simulink model "sim_elicottero_filtri"  (R2025b)
settings: Solver=ode4  StartTime=0.0  StopTime=15.0  FixedStep=0.001  RelTol=1e-3
values from neighbouring files (symbols this model uses):
  den_2nd = [1, 2*zeta*omega_n, omega_n^2]    [gen_dataset.m]
  den_pade = [tau_d/2, 1]    [gen_dataset.m]
  dt = log_vars.dt    [ekf_ukf.m]    (also in gen_dataset.m = 0.001)
  log_vars =     [EKF_smoother_data.mat]    (also in dataset_elicottero.mat)
  num_2nd = omega_n^2    (= 900)    [gen_dataset.m]
  num_pade = [-tau_d/2, 1]    [gen_dataset.m]
  p_hat = p    [gen_dataset.m]
  Q = diag([1e-5, 1e-3, 1e-5, 1e-3])    [ekf_ukf.m]    (also in gen_dataset.m = diag([)
  R = diag([0.05, 0.01])    [ekf_ukf.m]    (also in gen_dataset.m = diag([std_v_acc^2, std_v_mag^2, std_v_mag^2]))
  u_0 = [0; 0]    [gen_dataset.m]
  x_0 = [0.1; 0; 0.1; 0]    [gen_dataset.m]
libraries: simulink x4
settings Model: Creator=39345  LastModifiedBy=39345

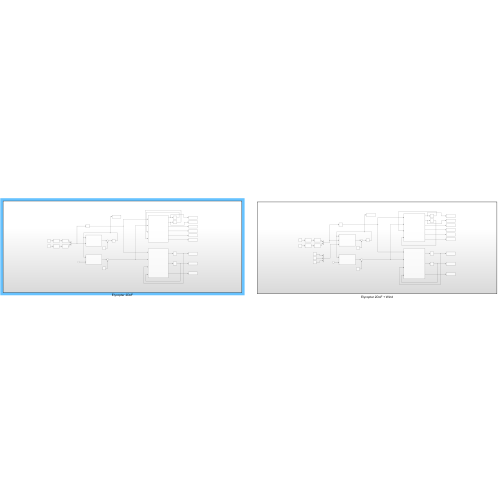
[thumbnail: Simulink's stored preview of the top-level diagram]
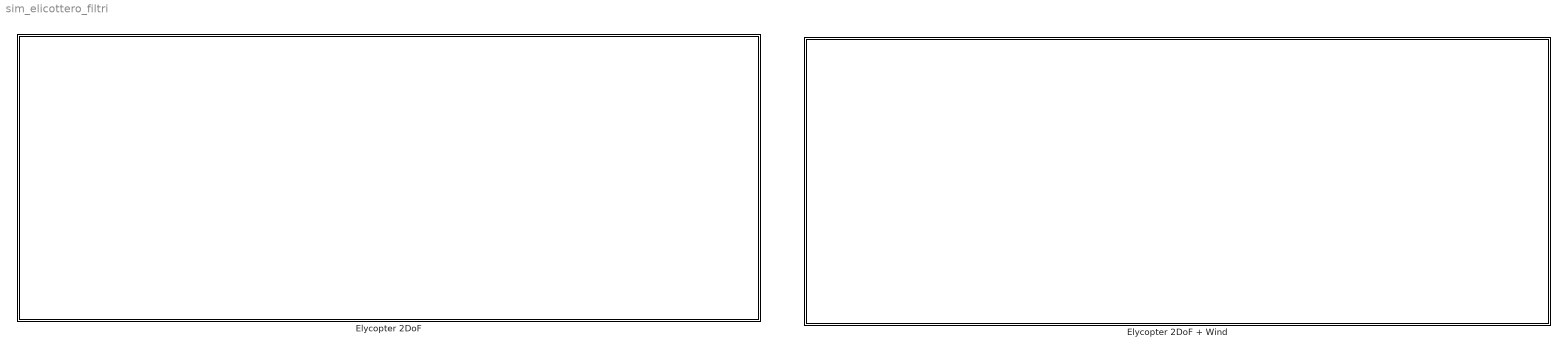
== system sim_elicottero_filtri ==
  Elycopter 2DoF : Subsystem
  Elycopter 2DoF + Wind : Subsystem

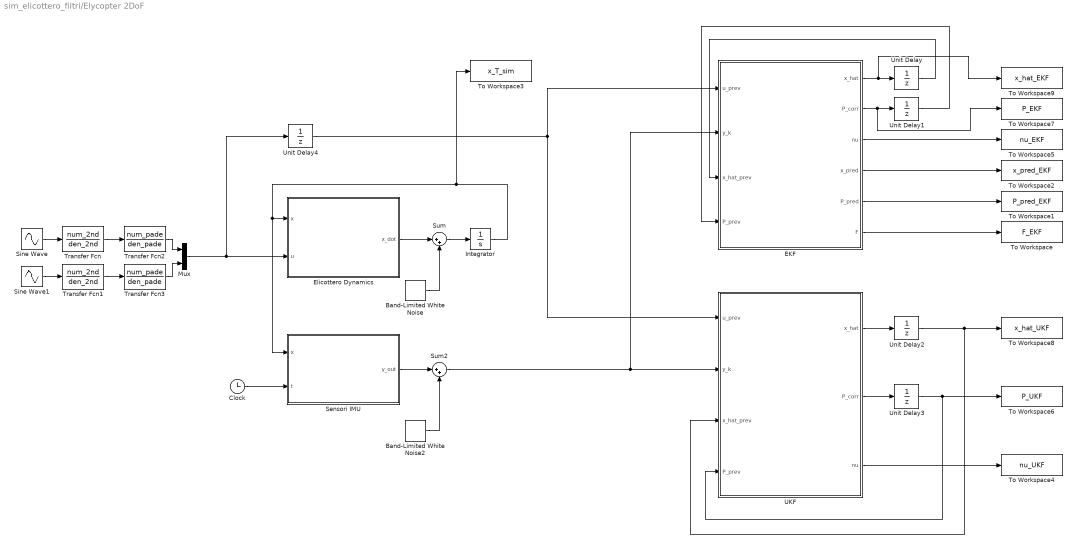
== system sim_elicottero_filtri/Elycopter 2DoF ==
  Band-Limited White Noise : simulink/Sources/Band-Limited White Noise  Cov=[0, 0.0025*dt, 0, 0.0025*dt]  Ts=dt  seed=[23341]
  Band-Limited White Noise2 : simulink/Sources/Band-Limited White Noise  Cov=[(0.2^2)*dt, (0.05^2)*0.01, (0.05^2)*0.01]  Ts=dt  seed=[23341]
  Clock : Clock
  EKF : MATLAB Function  TreatAsAtomicUnit=on
  Elicottero Dynamics : MATLAB Function  TreatAsAtomicUnit=on
  Integrator : Integrator  InitialCondition=x_0
  Mux : Mux  Inputs=2
  Sensori IMU : MATLAB Function  TreatAsAtomicUnit=on
  Sine Wave : Sin  Amplitude=0.5  Frequency=2  SampleTime=0
  Sine Wave1 : Sin  Amplitude=0.3  Frequency=1.5  Phase=pi/2  SampleTime=0
  Sum : Sum  Inputs=|++
  Sum2 : Sum  Inputs=|++
  To Workspace : ToWorkspace  VariableName=F_EKF  SaveFormat=Timeseries  SampleTime=-1
  To Workspace1 : ToWorkspace  VariableName=P_pred_EKF  SaveFormat=Timeseries  SampleTime=-1
  To Workspace2 : ToWorkspace  VariableName=x_pred_EKF  SaveFormat=Timeseries  SampleTime=-1
  To Workspace3 : ToWorkspace  VariableName=x_T_sim  SaveFormat=Timeseries  SampleTime=-1
  To Workspace4 : ToWorkspace  VariableName=nu_UKF  SaveFormat=Timeseries  SampleTime=-1
  To Workspace5 : ToWorkspace  VariableName=nu_EKF  SaveFormat=Timeseries  SampleTime=-1
  To Workspace6 : ToWorkspace  VariableName=P_UKF  SaveFormat=Timeseries  SampleTime=-1
  To Workspace7 : ToWorkspace  VariableName=P_EKF  SaveFormat=Timeseries  SampleTime=-1
  To Workspace8 : ToWorkspace  VariableName=x_hat_UKF  SaveFormat=Timeseries  SampleTime=-1
  To Workspace9 : ToWorkspace  VariableName=x_hat_EKF  SaveFormat=Timeseries  SampleTime=-1
  Transfer Fcn : TransferFcn  Numerator=num_2nd  Denominator=den_2nd
  Transfer Fcn1 : TransferFcn  Numerator=num_2nd  Denominator=den_2nd
  Transfer Fcn2 : TransferFcn  Numerator=num_pade  Denominator=den_pade
  Transfer Fcn3 : TransferFcn  Numerator=num_pade  Denominator=den_pade
  UKF : MATLAB Function  TreatAsAtomicUnit=on
  Unit Delay : UnitDelay  InitialCondition=log_vars.x_hat_0  SampleTime=-1  HasFrameUpgradeWarning=on
  Unit Delay1 : UnitDelay  InitialCondition=log_vars.P_0  SampleTime=dt  HasFrameUpgradeWarning=on
  Unit Delay2 : UnitDelay  InitialCondition=log_vars.x_hat_0  SampleTime=-1  HasFrameUpgradeWarning=on
  Unit Delay3 : UnitDelay  InitialCondition=log_vars.P_0  SampleTime=dt  HasFrameUpgradeWarning=on
  Unit Delay4 : UnitDelay  InitialCondition=u_0  SampleTime=dt  HasFrameUpgradeWarning=on
  wires:
  Sine Wave1/1 -> Transfer Fcn1/1
  UKF/2(P_corr) -> Unit Delay3/1
  EKF/5(P_pred) -> To Workspace1/1
  EKF/4(x_pred) -> To Workspace2/1
  Unit Delay2/1 -> To Workspace8/1, UKF/3(x_hat_prev)
  Transfer Fcn1/1 -> Transfer Fcn3/1
  Integrator/1 -> To Workspace3/1, Sensori IMU/1(x), Elicottero Dynamics/1(x)
  Mux/1 -> Unit Delay4/1, Elicottero Dynamics/2(u)
  Unit Delay3/1 -> To Workspace6/1, UKF/4(P_prev)
  Band-Limited White Noise2/1 -> Sum2/2
  UKF/3(nu) -> To Workspace4/1
  Unit Delay/1 -> EKF/3(x_hat_prev)
  Sum2/1 -> EKF/2(y_k), UKF/2(y_k)
  Sensori IMU/1(y_out) -> Sum2/1
  Unit Delay4/1 -> EKF/1(u_prev), UKF/1(u_prev)
  Transfer Fcn/1 -> Transfer Fcn2/1
  Transfer Fcn3/1 -> Mux/2
  Transfer Fcn2/1 -> Mux/1
  Unit Delay1/1 -> EKF/4(P_prev)
  EKF/6(F) -> To Workspace/1
  Band-Limited White Noise/1 -> Sum/2
  Elicottero Dynamics/1(x_dot) -> Sum/1
  EKF/2(P_corr) -> To Workspace7/1, Unit Delay1/1
  Sine Wave/1 -> Transfer Fcn/1
  EKF/3(nu) -> To Workspace5/1
  EKF/1(x_hat) -> To Workspace9/1, Unit Delay/1
  UKF/1(x_hat) -> Unit Delay2/1
  Sum/1 -> Integrator/1
  Clock/1 -> Sensori IMU/2(t)

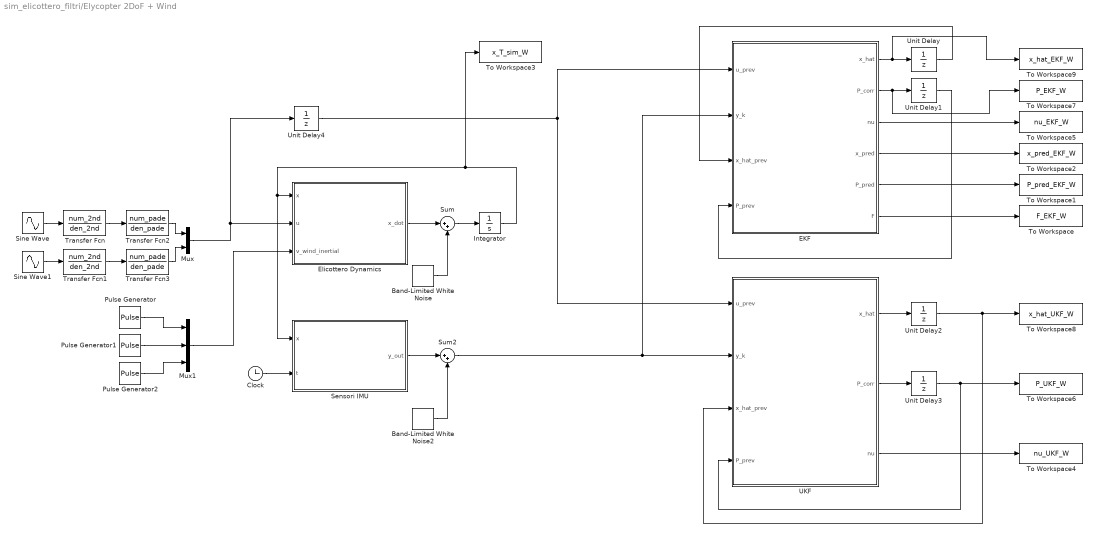
== system sim_elicottero_filtri/Elycopter 2DoF + Wind ==
  Band-Limited White Noise : simulink/Sources/Band-Limited White Noise  Cov=[0, 0.0025*dt, 0, 0.0025*dt]  Ts=dt  seed=[23341]
  Band-Limited White Noise2 : simulink/Sources/Band-Limited White Noise  Cov=[(0.2^2)*dt, (0.05^2)*0.01, (0.05^2)*0.01]  Ts=dt  seed=[23341]
  Clock : Clock
  EKF : MATLAB Function  TreatAsAtomicUnit=on
  Elicottero Dynamics : MATLAB Function  TreatAsAtomicUnit=on
  Integrator : Integrator  InitialCondition=x_0
  Mux : Mux  Inputs=2
  Mux1 : Mux  Inputs=3
  Pulse Generator : DiscretePulseGenerator  Period=10  PulseWidth=5  PhaseDelay=5
  Pulse Generator1 : DiscretePulseGenerator  Period=10  PulseWidth=5  PhaseDelay=5
  Pulse Generator2 : DiscretePulseGenerator  Period=10  PulseWidth=5  PhaseDelay=5
  Sensori IMU : MATLAB Function  TreatAsAtomicUnit=on
  Sine Wave : Sin  Amplitude=0.5  Frequency=2  SampleTime=0
  Sine Wave1 : Sin  Amplitude=0.3  Frequency=1.5  Phase=pi/2  SampleTime=0
  Sum : Sum  Inputs=|++
  Sum2 : Sum  Inputs=|++
  To Workspace : ToWorkspace  VariableName=F_EKF_W  SaveFormat=Timeseries  SampleTime=-1
  To Workspace1 : ToWorkspace  VariableName=P_pred_EKF_W  SaveFormat=Timeseries  SampleTime=-1
  To Workspace2 : ToWorkspace  VariableName=x_pred_EKF_W  SaveFormat=Timeseries  SampleTime=-1
  To Workspace3 : ToWorkspace  VariableName=x_T_sim_W  SaveFormat=Timeseries  SampleTime=-1
  To Workspace4 : ToWorkspace  VariableName=nu_UKF_W  SaveFormat=Timeseries  SampleTime=-1
  To Workspace5 : ToWorkspace  VariableName=nu_EKF_W  SaveFormat=Timeseries  SampleTime=-1
  To Workspace6 : ToWorkspace  VariableName=P_UKF_W  SaveFormat=Timeseries  SampleTime=-1
  To Workspace7 : ToWorkspace  VariableName=P_EKF_W  SaveFormat=Timeseries  SampleTime=-1
  To Workspace8 : ToWorkspace  VariableName=x_hat_UKF_W  SaveFormat=Timeseries  SampleTime=-1
  To Workspace9 : ToWorkspace  VariableName=x_hat_EKF_W  SaveFormat=Timeseries  SampleTime=-1
  Transfer Fcn : TransferFcn  Numerator=num_2nd  Denominator=den_2nd
  Transfer Fcn1 : TransferFcn  Numerator=num_2nd  Denominator=den_2nd
  Transfer Fcn2 : TransferFcn  Numerator=num_pade  Denominator=den_pade
  Transfer Fcn3 : TransferFcn  Numerator=num_pade  Denominator=den_pade
  UKF : MATLAB Function  TreatAsAtomicUnit=on
  Unit Delay : UnitDelay  InitialCondition=log_vars.x_hat_0  SampleTime=-1  HasFrameUpgradeWarning=on
  Unit Delay1 : UnitDelay  InitialCondition=log_vars.P_0  SampleTime=dt  HasFrameUpgradeWarning=on
  Unit Delay2 : UnitDelay  InitialCondition=log_vars.x_hat_0  SampleTime=-1  HasFrameUpgradeWarning=on
  Unit Delay3 : UnitDelay  InitialCondition=log_vars.P_0  SampleTime=dt  HasFrameUpgradeWarning=on
  Unit Delay4 : UnitDelay  InitialCondition=u_0  SampleTime=dt  HasFrameUpgradeWarning=on
  wires:
  Sine Wave1/1 -> Transfer Fcn1/1
  UKF/2(P_corr) -> Unit Delay3/1
  EKF/5(P_pred) -> To Workspace1/1
  EKF/4(x_pred) -> To Workspace2/1
  Unit Delay2/1 -> To Workspace8/1, UKF/3(x_hat_prev)
  Transfer Fcn1/1 -> Transfer Fcn3/1
  Integrator/1 -> To Workspace3/1, Sensori IMU/1(x), Elicottero Dynamics/1(x)
  Mux/1 -> Unit Delay4/1, Elicottero Dynamics/2(u)
  Unit Delay3/1 -> To Workspace6/1, UKF/4(P_prev)
  Band-Limited White Noise2/1 -> Sum2/2
  UKF/3(nu) -> To Workspace4/1
  Unit Delay/1 -> EKF/3(x_hat_prev)
  Sum2/1 -> EKF/2(y_k), UKF/2(y_k)
  Sensori IMU/1(y_out) -> Sum2/1
  Unit Delay4/1 -> EKF/1(u_prev), UKF/1(u_prev)
  Transfer Fcn/1 -> Transfer Fcn2/1
  Transfer Fcn3/1 -> Mux/2
  Transfer Fcn2/1 -> Mux/1
  Unit Delay1/1 -> EKF/4(P_prev)
  EKF/6(F) -> To Workspace/1
  Band-Limited White Noise/1 -> Sum/2
  Elicottero Dynamics/1(x_dot) -> Sum/1
  EKF/2(P_corr) -> To Workspace7/1, Unit Delay1/1
  Sine Wave/1 -> Transfer Fcn/1
  EKF/3(nu) -> To Workspace5/1
  EKF/1(x_hat) -> To Workspace9/1, Unit Delay/1
  UKF/1(x_hat) -> Unit Delay2/1
  Sum/1 -> Integrator/1
  Mux1/1 -> Elicottero Dynamics/3(v_wind_inertial)
  Pulse Generator/1 -> Mux1/1
  Pulse Generator1/1 -> Mux1/2
  Pulse Generator2/1 -> Mux1/3
  Clock/1 -> Sensori IMU/2(t)

== matlab function sim_elicottero_filtri/Elycopter 2DoF + Wind/Sensori IMU ==
  data: x input; y_out output; p parameter; t input
function y_out = sensori_imu(x, p, t)
    % ESTRAZIONE STATI RILEVANTI
    alpha = x(1);
    beta = x(3);
    
    % EQUAZIONI DEI SENSORI (Misure ideali)
    % 1. Accelerometro asse X (misura per alpha)
    y_acc = -p.g * sin(alpha);
    
    % 2. Magnetometro asse X e Y (misura per beta)
    mx = cos(alpha)*cos(beta);
    my = -sin(beta);

    y_out = [y_acc;
            mx;
            my];
    
    % ========================================================
    % LOGICA MULTI-RATE (Mascheramento dati mancanti)
    % ========================================================
    % Supponiamo che l'accelerometro (y_acc) lavori ad alta frequenza 
    % e sia sempre disponibile (quindi non lo tocchiamo).
    % Supponiamo che il magnetometro (y_mag) lavori a 10 Hz (un dato ogni 0.1 s).
    
    Tc_mag = 0.01; % Tempo di campionamento del sensore lento [secondi]
    tol = 1e-4;   % Tolleranza per gli arrotondamenti numerici di Simulink
    
    % Calcolo il resto della divisione tra il tempo attuale e il Tc del sensore
    resto = mod(t, Tc_mag);
    
    % Se il tempo attuale NON è un multiplo esatto di 0.1 secondi
    if resto > tol && (Tc_mag - resto) > tol
        % Il magnetometro non ha ancora prodotto un nuovo dato.
        % Sostituisco la seconda misura con Not a Number (NaN).
        y_out(2) = NaN; 
        y_out(3) = NaN;
    end
end

== matlab function sim_elicottero_filtri/Elycopter 2DoF + Wind/UKF ==
  data: u_prev input; x_hat output; y_k input; x_hat_prev input; P_prev input; P_corr output; nu output; Q parameter; R parameter; dt parameter; p_hat parameter
function [x_hat, P_corr, nu] = UKF_Filter(u_prev, y_k, x_hat_prev, P_prev, Q, R, dt, p_hat)
    
    % 1. Predizione UKF
    [x_pred, P_pred] = UnscentedTransform_F(x_hat_prev, P_prev, Q, dt, u_prev, p_hat);
    
    % 2. Correzione UKF
    [hat_y, S, Pxy] = UnscentedTransform_H(x_pred, P_pred, R, p_hat);
    
    % Logica Multi-rate
    idx_validi = ~isnan(y_k); 
    
    % Inizializzo default (come nell'EKF)
    x_hat = x_pred;
    P_corr = P_pred;
    nu = [0; 0; 0];
    
    if any(idx_validi)
        % Ritaglio solo i dati dei sensori attivi
        y_k_valid   = y_k(idx_validi);
        hat_y_valid = hat_y(idx_validi);
        
        S_valid   = S(idx_validi, idx_validi);
        Pxy_valid = Pxy(:, idx_validi); % Mantengo tutte le righe degli stati, ritaglio le colonne
        
        
        nu_valid = y_k_valid - hat_y_valid;
        
        % Salvo l'innovazione per i log
        nu(idx_validi) = nu_valid;

        % 3. DISTANZA DI MAHALANOBIS (Gating)
        D2 = nu_valid' * (S_valid \ nu_valid); 
        
        % Imposto la soglia Chi-Quadro al 95% in base a quanti sensori stanno parlando
        gradi_liberta = sum(idx_validi);
        if gradi_liberta == 1
            soglia = 3.84;
        else
            soglia = 7.81;
        end
        
        % 4. Aggiornamento dello Stato (solo se la misura è plausibile)
        if D2 < soglia
            L = Pxy_valid / S_valid;
            x_hat = x_pred + L * nu_valid;
            P_corr = P_pred - L * S_valid * L';            
        else
            % Outlier rilevato dal Mahalanobis! Ignoro la misura e tengo la predizione
            % (x_hat e P_corr restano x_pred e P_pred come inizializzato sopra)
        end
    end
end

% --- Funzioni Locali ---
function [mean_f, cov_f] = UnscentedTransform_F(x, P, Q, dt, u, p_hat)
    n = length(x);
    alpha = 1e-2; kappa = 0; beta = 2;
    lambda = alpha^2 * (n + kappa) - n;
    w_m = [lambda/(n+lambda), repmat(1/(2*(n+lambda)), 1, 2*n)];
    w_c = w_m; w_c(1) = w_c(1) + (1 - alpha^2 + beta);
    
    [U, S_mat, ~] = svd(P);
    GAMMA = U * sqrt(S_mat);
    
    sigmas = zeros(n, 2*n+1);
    sigmas(:,1) = x;
    for i = 1:n
        sigmas(:, i+1)   = x + sqrt(n+lambda)*GAMMA(:,i);
        sigmas(:, i+1+n) = x - sqrt(n+lambda)*GAMMA(:,i);
    end
    
    sigmas_f = zeros(n, 2*n+1);
    for i = 1:size(sigmas, 2)
        al = sigmas(1,i); al_d = sigmas(2,i); be = sigmas(3,i); be_d = sigmas(4,i);
        J_b = p_hat.J_y * sin(al)^2 + (p_hat.J_z + p_hat.m*p_hat.l^2)*cos(al)^2 + p_hat.I_b;

        % 1. Velocità angolare in Body
        omega_body = [-be_d * sin(al); al_d; be_d * cos(al)];
        % 2. Velocità lineare del corpo (v = omega x r)
        v_body = cross(omega_body, [p_hat.l; 0; 0]);
        % 3. Velocità relativa (il filtro assume vento esterno nullo)
        v_rel_body = -v_body;
        v_rel_norm = norm(v_rel_body);
        
        % 4. Forza aerodinamica (segno positivo corretto)
        F_drag_body = 0.5 * p_hat.rho * p_hat.Cd_A .* v_rel_body * v_rel_norm;
        
        % 5. Coppie di drag (segni corretti da prodotto vettoriale)
        tau_drag_alpha = -p_hat.l * F_drag_body(3);
        tau_drag_beta  =  p_hat.l * F_drag_body(2);

        al_dd = (-p_hat.c_alpha*al_d - p_hat.m*p_hat.g*p_hat.l*sin(al) + p_hat.l*u(1)*cos(be) + p_hat.eps_p*p_hat.l*u(2)*sin(be) + tau_drag_alpha) / p_hat.J_alpha;
        be_dd = (-p_hat.c_beta*be_d + p_hat.l*u(2)*cos(al) + p_hat.eps_y*p_hat.l*u(1)*sin(al) + tau_drag_beta) / J_b;
        sigmas_f(:,i) = [al + dt*al_d; al_d + dt*al_dd; be + dt*be_d; be_d + dt*be_dd];
    end
    
    mean_f = sigmas_f * w_m';
    tilde_f = sigmas_f - mean_f;
    cov_f = (tilde_f .* w_c) * tilde_f' + Q;
end

function [mean_h, cov_h, cross_cov] = UnscentedTransform_H(x, P, R, p_hat)
    n = length(x);
    alpha = 5e-2; kappa = 0; beta = 2;
    lambda = alpha^2 * (n + kappa) - n;
    
    w_m = [lambda/(n+lambda), repmat(1/(2*(n+lambda)), 1, 2*n)];
    w_c = w_m; w_c(1) = w_c(1) + (1 - alpha^2 + beta);
    
    [U, S_mat, ~] = svd(P);
    GAMMA = U * sqrt(S_mat);
    
    sigmas = zeros(n, 2*n+1);
    sigmas(:,1) = x;
    for i = 1:n
        sigmas(:, i+1)   = x + sqrt(n+lambda)*GAMMA(:,i);
        sigmas(:, i+1+n) = x - sqrt(n+lambda)*GAMMA(:,i);
    end
    
    sigmas_h = zeros(3, 2*n+1);
    for i = 1:size(sigmas, 2)
        sigmas_h(1,i) = -p_hat.g * sin(sigmas(1,i));
        sigmas_h(2,i) = cos(sigmas(1,i)) * cos(sigmas(3,i));
        sigmas_h(3,i) = -sin(sigmas(3,i));
    end
    
    mean_h = sigmas_h * w_m';
    tilde_h = sigmas_h - mean_h;
    cov_h = (tilde_h .* w_c) * tilde_h' + R;
    
    tilde_x = sigmas - x;
    cross_cov = (tilde_x .* w_c) * tilde_h';
end

== matlab function sim_elicottero_filtri/Elycopter 2DoF/Sensori IMU ==
  settings: sampleTime=dt
  data: x input; y_out output; p parameter; t input
function y_out = sensori_imu(x, p, t)
    % ESTRAZIONE STATI RILEVANTI
    alpha = x(1);
    beta = x(3);
    
    % EQUAZIONI DEI SENSORI (Misure ideali)
    % 1. Accelerometro asse X (misura per alpha)
    y_acc = -p.g * sin(alpha);
    
    % 2. Magnetometro asse X e Y (misura per beta)
    mx = cos(alpha)*cos(beta);
    my = -sin(beta);

    y_out = [y_acc;
            mx;
            my];
    
    % ========================================================
    % LOGICA MULTI-RATE (Mascheramento dati mancanti)
    % ========================================================
    % Supponiamo che l'accelerometro (y_acc) lavori ad alta frequenza 
    % e sia sempre disponibile (quindi non lo tocchiamo).
    % Supponiamo che il magnetometro (y_mag) lavori a 10 Hz (un dato ogni 0.1 s).
    
    Tc_mag = 0.01; % Tempo di campionamento del sensore lento [secondi]
    tol = 1e-4;   % Tolleranza per gli arrotondamenti numerici di Simulink
    
    % Calcolo il resto della divisione tra il tempo attuale e il Tc del sensore
    resto = mod(t, Tc_mag);
    
    % Se il tempo attuale NON è un multiplo esatto di 0.1 secondi
    if resto > tol && (Tc_mag - resto) > tol
        % Il magnetometro non ha ancora prodotto un nuovo dato.
        % Sostituisco la seconda misura con Not a Number (NaN).
        y_out(2) = NaN; 
        y_out(3) = NaN;
    end
end

== matlab function sim_elicottero_filtri/Elycopter 2DoF/Elicottero Dynamics ==
  data: x input; u input; x_dot output; p parameter
function x_dot = elicottero_dynamics(x, u, p)
    % ESTRAZIONE STATI
    alpha = x(1);
    alpha_dot = x(2);
    beta = x(3);
    beta_dot = x(4);
    
    % ESTRAZIONE INGRESSI
    F1 = u(1);
    F2 = u(2);
                 
    % 1. Vettore velocità angolare nel sistema Body (omega_B)
    % Il Pitch (alpha_dot) ruota attorno all'asse Y_body.
    % Lo Yaw (beta_dot) ruota attorno all'asse Z_inerziale, che proiettato in Body diventa [-sin(alpha); 0; cos(alpha)]
    omega_body = [-beta_dot * sin(alpha); 
                   alpha_dot; 
                   beta_dot * cos(alpha)];
                   
    % 2. Vettore posizione del centro aerodinamico (i rotori a distanza l sull'asse X_body)
    r_cp = [p.l; 0; 0];
    
    % 3. Velocità lineare del corpo dovuta alla rotazione (v = omega x r)
    v_corpo_body = cross(omega_body, r_cp); 
    % (Il risultato analitico sarà: [0; p.l * beta_dot * cos(alpha); -p.l * alpha_dot])
    
    
    % 5. VELOCITÀ RELATIVA VERA (Vento esterno - Velocità del corpo)
    v_rel_body  = - v_corpo_body; 
    v_rel_norm  = norm(v_rel_body);
    
    % Calcolo Forze Aerodinamiche
    % NOTA: Per pulizia del codice, in futuro potresti spostare rho e Cd_A 
    % all'interno della struct dei parametri 'p'
    rho = 1.225; % Densità dell'aria [kg/m^3]
    Cd_A = [0.1
            0.1
            0.2]; % Prodotto Cd * Area per gli assi [X; Y; Z]
    % Bracci da $0.25$ e $0.30$ m: Sono lunghezze tipiche dei bracci di un 
    % elicottero didattico da laboratorio a 2 gradi di libertà, come i 
    % classici modelli Quanser Aero o i TRMS (Twin Rotor MIMO System)
    
    F_drag_body = 0.5 * rho * Cd_A .* v_rel_body * v_rel_norm;
    
    % Calcolo Coppie di Disturbo
    % Assumiamo che la forza aerodinamica agisca con braccio pari a p.l
    tau_wind_alpha = -F_drag_body(3) * p.l; % Forza verticale genera coppia di pitch
    tau_wind_beta  = F_drag_body(2) * p.l; % Forza laterale genera coppia di yaw
    
    % DINAMICA: Inerzia variabile di yaw
    J_beta = p.J_y * sin(alpha)^2 + (p.J_z + p.m*p.l^2)*cos(alpha)^2 + p.I_b;
    
    % EQUAZIONI DEL MOTO (Accelerazioni)
    % I momenti del vento sono sommati ai momenti generati dai motori
    alpha_ddot = (-p.c_alpha*alpha_dot - p.m*p.g*p.l*sin(alpha) + p.l*F1*cos(beta) + p.eps_p*p.l*F2*sin(beta) + tau_wind_alpha) / p.J_alpha;
    beta_ddot  = (-p.c_beta*beta_dot + p.l*F2*cos(alpha) + p.eps_y*p.l*F1*sin(alpha) + tau_wind_beta) / J_beta;
    
    
    % USCITA: Vettore colonna delle derivate dello stato
    x_dot = [alpha_dot; alpha_ddot; beta_dot; beta_ddot];
end

== matlab function sim_elicottero_filtri/Elycopter 2DoF/EKF ==
  data: u_prev input; x_hat output; y_k input; x_hat_prev input; P_prev input; P_corr output; nu output; Q parameter; R parameter; dt parameter; p_hat parameter; x_pred output; P_pred output; F output
function [x_hat, P_corr, nu, x_pred, P_pred, F] = EKF_Filter(u_prev, y_k, x_hat_prev, P_prev, Q, R, dt, p_hat)
    % ========================================================
    % 1. FASE DI PREDIZIONE
    % ========================================================
    alpha = x_hat_prev(1); alpha_dot = x_hat_prev(2); 
    beta = x_hat_prev(3);  beta_dot = x_hat_prev(4);
    F1 = u_prev(1); F2 = u_prev(2);

    rho = 1.225; % Densità dell'aria [kg/m^3]
    Cd_A = [0.5; 0.6; 1.2]; % Prodotto Cd * Area per gli assi [X; Y; Z]
    
    J_beta = p_hat.J_y * sin(alpha)^2 + (p_hat.J_z + p_hat.m*p_hat.l^2)*cos(alpha)^2 + p_hat.I_b;

    omega_body = [-beta_dot * sin(alpha); alpha_dot; beta_dot * cos(alpha)];
    v_corpo_body = cross(omega_body, [p_hat.l; 0; 0]);
    v_rel_body = -v_corpo_body; % Il filtro assume vento esterno nullo
    v_rel_norm = norm(v_rel_body);
    
    F_drag_body = 0.5 * rho * Cd_A .* v_rel_body * v_rel_norm;
    tau_drag_alpha = -F_drag_body(3) * p_hat.l;
    tau_drag_beta  = F_drag_body(2) * p_hat.l;

    alpha_ddot = (-p_hat.c_alpha*alpha_dot - p_hat.m*p_hat.g*p_hat.l*sin(alpha) + p_hat.l*F1*cos(beta) + p_hat.eps_p*p_hat.l*F2*sin(beta) + tau_drag_alpha) / p_hat.J_alpha;
    beta_ddot  = (-p_hat.c_beta*beta_dot + p_hat.l*F2*cos(alpha) + p_hat.eps_y*p_hat.l*F1*sin(alpha) + tau_drag_beta) / J_beta;
    
    x_pred = [alpha + dt * alpha_dot;
              alpha_dot + dt * alpha_ddot;
              beta + dt * beta_dot;
              beta_dot + dt * beta_ddot];

    % Jacobiano numerico F
    [F, ~] = jacobiani_analitici(x_hat_prev(1), x_hat_prev(2), x_hat_prev(3), x_hat_prev(4), ...
                           u_prev(1), u_prev(2), dt, rho, ...
                           p_hat.m, p_hat.l, p_hat.g, p_hat.J_y, p_hat.J_z, p_hat.I_b, p_hat.J_alpha, ...
                           p_hat.c_alpha, p_hat.c_beta, p_hat.eps_p, p_hat.eps_y, ...
                           Cd_A(1), Cd_A(2), Cd_A(3));

    P_pred = F * P_prev * F' + Q;

% ========================================================
    % 2. FASE DI CORREZIONE
    % ========================================================
    % Calcolo la misura attesa completa
    hat_y = [-p_hat.g * sin(x_pred(1));
             cos(x_pred(1)) * cos(x_pred(3));
             -sin(x_pred(3))];
    
    % Calcolo il Jacobiano H completo
    [~, H] = jacobiani_analitici(x_pred(1), x_pred(2), x_pred(3), x_pred(4), ...
                           u_prev(1), u_prev(2), dt, rho, ...
                           p_hat.m, p_hat.l, p_hat.g, p_hat.J_y, p_hat.J_z, p_hat.I_b, p_hat.J_alpha, ...
                           p_hat.c_alpha, p_hat.c_beta, p_hat.eps_p, p_hat.eps_y, ...
                           Cd_A(1), Cd_A(2), Cd_A(3));
     
    % Trovo quali sensori hanno inviato un dato valido in questo istante
    % (idx_validi sarà un vettore logico, es: [1; 0] se è arrivato solo il sensore 1)
    idx_validi = ~isnan(y_k); 
    
    % Inizializzo le uscite di default (se nessun sensore parla, tengo la predizione)
    x_hat = x_pred;
    P_corr = P_pred;
    nu = [0; 0; 0]; % Innovazione nulla di default
    
    if any(idx_validi) % Se almeno un sensore ha un dato nuovo
        
        % 1. "RitAGLIO" i vettori e le matrici tenendo solo le righe dei sensori attivi
        y_k_valid   = y_k(idx_validi);
        hat_y_valid = hat_y(idx_validi);
        H_valid     = H(idx_validi, :);
        
        % Ritaglio anche la matrice R (rumore di misura) per togliere il sensore inattivo
        R_valid     = R(idx_validi, idx_validi);
        
        % 2. Calcolo Innovazione e Covarianza dell'Innovazione ridimensionate
        nu_valid = y_k_valid - hat_y_valid;
        S = H_valid * P_pred * H_valid' + R_valid;
        
        % 3. DISTANZA DI MAHALANOBIS (Gating)
        D2 = nu_valid' * (S \ nu_valid); 
        
        % Imposto la soglia Chi-Quadro al 95% in base a quanti sensori stanno parlando
        gradi_liberta = sum(idx_validi);
        if gradi_liberta == 1
            soglia = 3.84;
        else
            soglia = 5.99;
        end
        
        % 4. Aggiornamento dello Stato (solo se la misura è plausibile)
        if D2 < soglia
            L = P_pred * H_valid' / S;
            x_hat = x_pred + L * nu_valid;
            P_corr = (eye(4) - L * H_valid) * P_pred;
            
            % Salvo l'innovazione calcolata per i log (lasciando 0 dove mancava il dato)
            nu(idx_validi) = nu_valid; 
        else
            % Outlier rilevato dal Mahalanobis! Ignoro la misura e tengo la predizione
            % (x_hat e P_corr restano x_pred e P_pred come inizializzato sopra)
        end
        
    end
end

== matlab function sim_elicottero_filtri/Elycopter 2DoF/UKF ==
  data: u_prev input; x_hat output; y_k input; x_hat_prev input; P_prev input; P_corr output; nu output; Q parameter; R parameter; dt parameter; p_hat parameter
function [x_hat, P_corr, nu] = UKF_Filter(u_prev, y_k, x_hat_prev, P_prev, Q, R, dt, p_hat)
    
    % 1. Predizione UKF
    [x_pred, P_pred] = UnscentedTransform_F(x_hat_prev, P_prev, Q, dt, u_prev, p_hat);
    
    % 2. Correzione UKF
    [hat_y, S, Pxy] = UnscentedTransform_H(x_pred, P_pred, R, p_hat);
    
    % Logica Multi-rate
    idx_validi = ~isnan(y_k); 
    
    % Inizializzo default (come nell'EKF)
    x_hat = x_pred;
    P_corr = P_pred;
    nu = [0; 0; 0];
    
    if any(idx_validi)
        % Ritaglio solo i dati dei sensori attivi
        y_k_valid   = y_k(idx_validi);
        hat_y_valid = hat_y(idx_validi);
        
        S_valid   = S(idx_validi, idx_validi);
        Pxy_valid = Pxy(:, idx_validi); % Mantengo tutte le righe degli stati, ritaglio le colonne
        
        
        nu_valid = y_k_valid - hat_y_valid;
        
        % Salvo l'innovazione per i log
        nu(idx_validi) = nu_valid;

        % 3. DISTANZA DI MAHALANOBIS (Gating)
        D2 = nu_valid' * (S_valid \ nu_valid); 
        
        % Imposto la soglia Chi-Quadro al 95% in base a quanti sensori stanno parlando
        gradi_liberta = sum(idx_validi);
        if gradi_liberta == 1
            soglia = 3.84;
        else
            soglia = 7.81;
        end
        
        % 4. Aggiornamento dello Stato (solo se la misura è plausibile)
        if D2 < soglia
            L = Pxy_valid / S_valid;
            x_hat = x_pred + L * nu_valid;
            P_corr = P_pred - L * S_valid * L';            
        else
            % Outlier rilevato dal Mahalanobis! Ignoro la misura e tengo la predizione
            % (x_hat e P_corr restano x_pred e P_pred come inizializzato sopra)
        end
    end
end

% --- Funzioni Locali ---
function [mean_f, cov_f] = UnscentedTransform_F(x, P, Q, dt, u, p_hat)
    n = length(x);
    alpha = 1e-2; kappa = 0; beta = 2;
    lambda = alpha^2 * (n + kappa) - n;
    w = [0 0 0];
    w_m = [lambda/(n+lambda), repmat(1/(2*(n+lambda)), 1, 2*n)];
    w_c = w_m; w_c(1) = w_c(1) + (1 - alpha^2 + beta);
    
    [U, S_mat, ~] = svd(P);
    GAMMA = U * sqrt(S_mat);
    
    sigmas = zeros(n, 2*n+1);
    sigmas(:,1) = x;
    for i = 1:n
        sigmas(:, i+1)   = x + sqrt(n+lambda)*GAMMA(:,i);
        sigmas(:, i+1+n) = x - sqrt(n+lambda)*GAMMA(:,i);
    end
    
    sigmas_f = zeros(n, 2*n+1);
    for i = 1:size(sigmas, 2)
        al = sigmas(1,i); al_d = sigmas(2,i); be = sigmas(3,i); be_d = sigmas(4,i);
        J_b = p_hat.J_y * sin(al)^2 + (p_hat.J_z + p_hat.m*p_hat.l^2)*cos(al)^2 + p_hat.I_b;

        % 1. Velocità angolare in Body
        omega_body = [-be_d * sin(al); al_d; be_d * cos(al)];
        % 2. Velocità lineare del corpo (v = omega x r)
        v_body = cross(omega_body, [p_hat.l; 0; 0]);
        % 3. Velocità relativa (il filtro assume vento esterno nullo)
        v_rel_body = -v_body + w;
        v_rel_norm = norm(v_rel_body);
        
        % 4. Forza aerodinamica (segno positivo corretto)
        F_drag_body = 0.5 * p_hat.rho * p_hat.Cd_A .* v_rel_body * v_rel_norm;
        
        % 5. Coppie di drag (segni corretti da prodotto vettoriale)
        tau_drag_alpha = -p_hat.l * F_drag_body(3);
        tau_drag_beta  =  p_hat.l * F_drag_body(2);

        al_dd = (-p_hat.c_alpha*al_d - p_hat.m*p_hat.g*p_hat.l*sin(al) + p_hat.l*u(1)*cos(be) + p_hat.eps_p*p_hat.l*u(2)*sin(be) + tau_drag_alpha) / p_hat.J_alpha;
        be_dd = (-p_hat.c_beta*be_d + p_hat.l*u(2)*cos(al) + p_hat.eps_y*p_hat.l*u(1)*sin(al) + tau_drag_beta) / J_b;
        sigmas_f(:,i) = [al + dt*al_d; al_d + dt*al_dd; be + dt*be_d; be_d + dt*be_dd];
    end
    
    mean_f = sigmas_f * w_m';
    tilde_f = sigmas_f - mean_f;
    cov_f = (tilde_f .* w_c) * tilde_f' + Q;
end

function [mean_h, cov_h, cross_cov] = UnscentedTransform_H(x, P, R, p_hat)
    n = length(x);
    alpha = 5e-2; kappa = 0; beta = 2;
    lambda = alpha^2 * (n + kappa) - n;
    
    w_m = [lambda/(n+lambda), repmat(1/(2*(n+lambda)), 1, 2*n)];
    w_c = w_m; w_c(1) = w_c(1) + (1 - alpha^2 + beta);
    
    [U, S_mat, ~] = svd(P);
    GAMMA = U * sqrt(S_mat);
    
    sigmas = zeros(n, 2*n+1);
    sigmas(:,1) = x;
    for i = 1:n
        sigmas(:, i+1)   = x + sqrt(n+lambda)*GAMMA(:,i);
        sigmas(:, i+1+n) = x - sqrt(n+lambda)*GAMMA(:,i);
    end
    
    sigmas_h = zeros(3, 2*n+1);
    for i = 1:size(sigmas, 2)
        sigmas_h(1,i) = -p_hat.g * sin(sigmas(1,i));
        sigmas_h(2,i) = cos(sigmas(1,i)) * cos(sigmas(3,i));
        sigmas_h(3,i) = -sin(sigmas(3,i));
    end
    
    mean_h = sigmas_h * w_m';
    tilde_h = sigmas_h - mean_h;
    cov_h = (tilde_h .* w_c) * tilde_h' + R;
    
    tilde_x = sigmas - x;
    cross_cov = (tilde_x .* w_c) * tilde_h';
end

== matlab function sim_elicottero_filtri/Elycopter 2DoF + Wind/EKF ==
  data: u_prev input; x_hat output; y_k input; x_hat_prev input; P_prev input; P_corr output; nu output; Q parameter; R parameter; dt parameter; p_hat parameter; x_pred output; P_pred output; F output
function [x_hat, P_corr, nu, x_pred, P_pred, F] = EKF_Filter(u_prev, y_k, x_hat_prev, P_prev, Q, R, dt, p_hat)
    % ========================================================
    % 1. FASE DI PREDIZIONE (predict_EKF)
    % ========================================================
    alpha = x_hat_prev(1); alpha_dot = x_hat_prev(2); 
    beta = x_hat_prev(3);  beta_dot = x_hat_prev(4);
    F1 = u_prev(1); F2 = u_prev(2);

    rho = 1.225; % Densità dell'aria [kg/m^3]
    Cd_A = [0.5; 0.6; 1.2]; % Prodotto Cd * Area per gli assi [X; Y; Z]
    J_beta = p_hat.J_y * sin(alpha)^2 + (p_hat.J_z + p_hat.m*p_hat.l^2)*cos(alpha)^2 + p_hat.I_b;

    omega_body = [-beta_dot * sin(alpha); alpha_dot; beta_dot * cos(alpha)];
    v_body = cross(omega_body, [p_hat.l; 0; 0]);
    v_rel_body = -v_body; % Il filtro assume vento esterno nullo
    v_rel_norm = norm(v_rel_body);
    
    F_drag_body = 0.5 * rho * Cd_A .* v_rel_body * v_rel_norm;
    tau_drag_alpha = -F_drag_body(3) * p_hat.l;
    tau_drag_beta  = F_drag_body(2) * p_hat.l;

    alpha_ddot = (-p_hat.c_alpha*alpha_dot - p_hat.m*p_hat.g*p_hat.l*sin(alpha) + p_hat.l*F1*cos(beta) + p_hat.eps_p*p_hat.l*F2*sin(beta) + tau_drag_alpha) / p_hat.J_alpha;
    beta_ddot  = (-p_hat.c_beta*beta_dot + p_hat.l*F2*cos(alpha) + p_hat.eps_y*p_hat.l*F1*sin(alpha) + tau_drag_beta) / J_beta;
    
    x_pred = [alpha + dt * alpha_dot;
              alpha_dot + dt * alpha_ddot;
              beta + dt * beta_dot;
              beta_dot + dt * beta_ddot];

    % Jacobiano numerico F
    [F, ~] = jacobiani_analitici(x_hat_prev(1), x_hat_prev(2), x_hat_prev(3), x_hat_prev(4), ...
                           u_prev(1), u_prev(2), dt, rho, ...
                           p_hat.m, p_hat.l, p_hat.g, p_hat.J_y, p_hat.J_z, p_hat.I_b, p_hat.J_alpha, ...
                           p_hat.c_alpha, p_hat.c_beta, p_hat.eps_p, p_hat.eps_y, ...
                           Cd_A(1), Cd_A(2), Cd_A(3));

    P_pred = F * P_prev * F' + Q;

    % ========================================================
    % 2. FASE DI CORREZIONE (correct_EKF) - MULTI-RATE
    % ========================================================
    % Calcolo la misura attesa completa
    hat_y = [-p_hat.g * sin(x_pred(1));
             cos(x_pred(1)) * cos(x_pred(3));
             -sin(x_pred(3))];
    
    % Calcolo il Jacobiano H completo
    [~, H] = jacobiani_analitici(x_pred(1), x_pred(2), x_pred(3), x_pred(4), ...
                           u_prev(1), u_prev(2), dt, rho, ...
                           p_hat.m, p_hat.l, p_hat.g, p_hat.J_y, p_hat.J_z, p_hat.I_b, p_hat.J_alpha, ...
                           p_hat.c_alpha, p_hat.c_beta, p_hat.eps_p, p_hat.eps_y, ...
                           Cd_A(1), Cd_A(2), Cd_A(3));
     
    % Trovo quali sensori hanno inviato un dato valido in questo istante
    % (idx_validi sarà un vettore logico, es: [1; 0] se è arrivato solo il sensore 1)
    idx_validi = ~isnan(y_k); 
    
    % Inizializzo le uscite di default (se nessun sensore parla, tengo la predizione)
    x_hat = x_pred;
    P_corr = P_pred;
    nu = [0; 0; 0]; % Innovazione nulla di default
    
    if any(idx_validi) % Se almeno un sensore ha un dato nuovo
        
        % 1. "Ritaglio" i vettori e le matrici tenendo solo le righe dei sensori attivi
        y_k_valid   = y_k(idx_validi);
        hat_y_valid = hat_y(idx_validi);
        H_valid     = H(idx_validi, :);
        
        % Ritaglio anche la matrice R (rumore di misura) per togliere il sensore inattivo
        R_valid     = R(idx_validi, idx_validi);
        
        % 2. Calcolo Innovazione e Covarianza dell'Innovazione ridimensionate
        nu_valid = y_k_valid - hat_y_valid;
        S = H_valid * P_pred * H_valid' + R_valid;
        
        % 3. DISTANZA DI MAHALANOBIS (Gating)
        D2 = nu_valid' * (S \ nu_valid); 
        
        % Imposto la soglia Chi-Quadro al 95% in base a quanti sensori stanno parlando
        gradi_liberta = sum(idx_validi);
        if gradi_liberta == 1
            soglia = 3.84;
        else
            soglia = 5.99;
        end
        
        % 4. Aggiornamento dello Stato (solo se la misura è plausibile)
        if D2 < soglia
            L = P_pred * H_valid' / S;
            x_hat = x_pred + L * nu_valid;
            P_corr = (eye(4) - L * H_valid) * P_pred;
            
            % Salvo l'innovazione calcolata per i log (lasciando 0 dove mancava il dato)
            nu(idx_validi) = nu_valid; 
        else
            % Outlier rilevato dal Mahalanobis! Ignoro la misura e tengo la predizione
            % (x_hat e P_corr restano x_pred e P_pred come inizializzato sopra)
        end
        
    end
end

== matlab function sim_elicottero_filtri/Elycopter 2DoF + Wind/Elicottero Dynamics ==
  data: x input; u input; x_dot output; p parameter; v_wind_inertial input
function x_dot = elicottero_dynamics(x, u, p, v_wind_inertial)
    % ESTRAZIONE STATI
    alpha = x(1);
    alpha_dot = x(2);
    beta = x(3);
    beta_dot = x(4);
    
    % ESTRAZIONE INGRESSI
    F1 = u(1);
    F2 = u(2);
    
    % Matrice di rotazione da Inerziale a Body (Roll = 0)
    % Usiamo alpha per il Pitch e beta per lo Yaw
    R_I_to_B = [ cos(alpha)*cos(beta),  cos(alpha)*sin(beta), -sin(alpha);
                         -sin(beta),              cos(beta),            0;
                 sin(alpha)*cos(beta),  sin(alpha)*sin(beta),  cos(alpha) ];
                 
    % 1. Vettore velocità angolare nel sistema Body (omega_B)
    % Il Pitch (alpha_dot) ruota attorno all'asse Y_body.
    % Lo Yaw (beta_dot) ruota attorno all'asse Z_inerziale, che proiettato in Body diventa [-sin(alpha); 0; cos(alpha)]
    omega_body = [-beta_dot * sin(alpha); 
                   alpha_dot; 
                   beta_dot * cos(alpha)];
                   
    % 2. Vettore posizione del centro aerodinamico (i rotori a distanza l sull'asse X_body)
    r_cp = [p.l; 0; 0];
    
    % 3. Velocità lineare del corpo dovuta alla rotazione (v = omega x r)
    v_corpo_body = cross(omega_body, r_cp); 
    % (Il risultato analitico sarà: [0; p.l * beta_dot * cos(alpha); -p.l * alpha_dot])
    
    % 4. Vento esterno nel sistema Body
    v_wind_body = R_I_to_B * v_wind_inertial;
    
    % 5. VELOCITÀ RELATIVA VERA (Vento esterno - Velocità del corpo)
    v_rel_body  = v_wind_body - v_corpo_body; 
    v_rel_norm  = norm(v_rel_body);
    
    % Calcolo Forze Aerodinamiche
    % all'interno della struct dei parametri 'p'
    rho = 1.225; % Densità dell'aria [kg/m^3]
    Cd_A = [0.1
            0.1
            0.2]; % Prodotto Cd * Area per gli assi [X; Y; Z]
    % Bracci da $0.25$ e $0.30$ m: Sono lunghezze tipiche dei bracci di un 
    % elicottero didattico da laboratorio a 2 gradi di libertà, come i 
    % classici modelli Quanser Aero o i TRMS (Twin Rotor MIMO System)
    
    F_drag_body = 0.5 * rho * Cd_A .* v_rel_body * v_rel_norm;
    
    % Calcolo Coppie di Disturbo
    % Assumiamo che la forza aerodinamica agisca con braccio pari a p.l
    tau_wind_alpha = -F_drag_body(3) * p.l; % Forza verticale genera coppia di pitch
    tau_wind_beta  = F_drag_body(2) * p.l; % Forza laterale genera coppia di yaw
    
    % DINAMICA: Inerzia variabile di yaw
    J_beta = p.J_y * sin(alpha)^2 + (p.J_z + p.m*p.l^2)*cos(alpha)^2 + p.I_b;
    
    % EQUAZIONI DEL MOTO (Accelerazioni)
    % I momenti del vento sono sommati ai momenti generati dai motori
    alpha_ddot = (-p.c_alpha*alpha_dot - p.m*p.g*p.l*sin(alpha) + p.l*F1*cos(beta) + p.eps_p*p.l*F2*sin(beta) + tau_wind_alpha) / p.J_alpha;
    beta_ddot  = (-p.c_beta*beta_dot + p.l*F2*cos(alpha) + p.eps_y*p.l*F1*sin(alpha) + tau_wind_beta) / J_beta;
    
    
    % USCITA: Vettore colonna delle derivate dello stato
    x_dot = [alpha_dot; alpha_ddot; beta_dot; beta_ddot];
end
